simulink model "SimForKid"  (R2019b)
settings: Solver=ode23  StartTime=0.0  StopTime=30  FixedStep=1e-6  RelTol=1e-7
libraries: dsparch4 x3
settings Model: Creator=19398  LastModifiedBy=19398

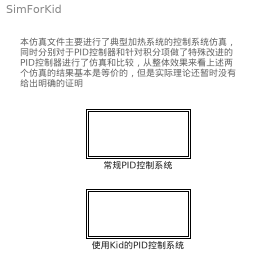
== system SimForKid ==
  note: 本仿真文件主要进行了典型加热系统的控制系统仿真，
      | 同时分别对于PID控制器和针对积分项做了特殊改进的
      | PID控制器进行了仿真和比较，从整体效果来看上述两
      | 个仿真的结果基本是等价的，但是实际理论还暂时没有
      | 给出明确的证明
  使用Kid的PID控制系统 : Subsystem
  常规PID控制系统 : Subsystem

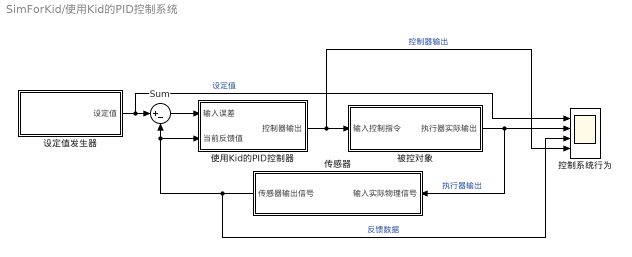
== system SimForKid/使用Kid的PID控制系统 ==
  Sum : Sum  Inputs=|+-
  传感器 : Subsystem
  使用Kid的PID控制器 : Subsystem  mask{Kp=50, Ki=0.5, iLimit=300, Kid=2, Kd=200, c=500, DFilterOrder=6, DFilterFreq=300, OutLim=75}
      mask prompts: Kp "比例增益系数"; Ki "积分增益系数"; iLimit "积分限幅"; Kid "积分微分增益"; Kd "微分增益系数"; c "实际微分系数"; DFilterOrder "微分滤波器阶数"; DFilterFreq "微分滤波器截止频率Hz"; OutLim "输出限幅"
  控制系统行为 : Scope  NumInputPorts=4
  被控对象 : Subsystem
  设定值发生器 : Subsystem
  wires:
  使用Kid的PID控制器/1(控制器输出) -> 控制系统行为/4, 被控对象/1(输入控制指令)  "控制器输出"
  设定值发生器/1(设定值) -> 控制系统行为/1, Sum/1  "设定值"
  被控对象/1(执行器实际输出) -> 控制系统行为/2, 传感器/1(输入实际物理信号)  "执行器输出"
  Sum/1 -> 使用Kid的PID控制器/1(输入误差)
  传感器/1(传感器输出信号) -> 控制系统行为/3, 使用Kid的PID控制器/2(当前反馈值), Sum/2  "反馈数据"

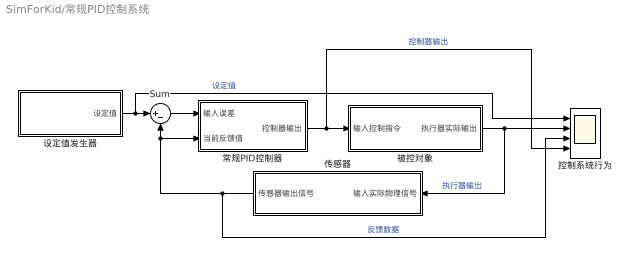
== system SimForKid/常规PID控制系统 ==
  Sum : Sum  Inputs=|+-
  传感器 : Subsystem
  常规PID控制器 : Subsystem  mask{Kp=50, Ki=0.2, iLimit=300, Kd=200, c=500, DFilterOrder=6, DFilterFreq=300, OutLim=75}
      mask prompts: Kp "比例增益系数"; Ki "积分增益系数"; iLimit "积分限幅"; Kd "微分增益系数"; c "实际微分系数"; DFilterOrder "微分滤波器阶数"; DFilterFreq "微分滤波器截止频率Hz"; OutLim "输出限幅"
  控制系统行为 : Scope  NumInputPorts=4
  被控对象 : Subsystem
  设定值发生器 : Subsystem
  wires:
  常规PID控制器/1(控制器输出) -> 控制系统行为/4, 被控对象/1(输入控制指令)  "控制器输出"
  设定值发生器/1(设定值) -> 控制系统行为/1, Sum/1  "设定值"
  被控对象/1(执行器实际输出) -> 控制系统行为/2, 传感器/1(输入实际物理信号)  "执行器输出"
  Sum/1 -> 常规PID控制器/1(输入误差)
  传感器/1(传感器输出信号) -> 控制系统行为/3, 常规PID控制器/2(当前反馈值), Sum/2  "反馈数据"

== system SimForKid/使用Kid的PID控制系统/传感器 ==
  输入实际物理信号 : Inport
  传感滞后 : TransferFcn  Denominator=[6 1]
  通信延迟 : TransportDelay  DelayTime=0.001
  传感器输出信号 : Outport
  wires:
  传感滞后/1 -> 通信延迟/1
  通信延迟/1 -> 传感器输出信号/1
  输入实际物理信号/1 -> 传感滞后/1

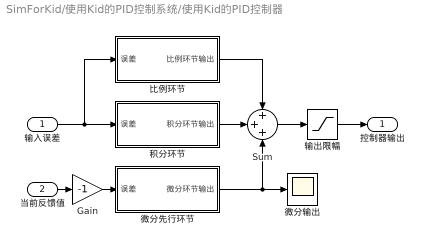
== system SimForKid/使用Kid的PID控制系统/使用Kid的PID控制器 ==
  输入误差 : Inport
  当前反馈值 : Inport  Port=2
  Gain : Gain  Gain=-1
  Sum : Sum  Inputs=+++
  微分先行环节 : Subsystem  mask{Kd=Kd, c=c, DFilterOrder=DFilterOrder, DFilterFreq=DFilterFreq}
      mask prompts: Kd "微分增益系数"; c "实际微分系数"; DFilterOrder "微分滤波器阶数"; DFilterFreq "微分滤波器截止频率Hz"
  微分输出 : Scope
  比例环节 : Subsystem  mask{Kp=Kp}
      mask prompts: Kp "比例增益系数"
  积分环节 : Subsystem  mask{Ki=Ki, iLimit=iLimit, Kid=Kid}
      mask prompts: Ki "积分增益系数"; iLimit "积分限幅"; Kid "积分微分增益"
  输出限幅 : Saturate  UpperLimit=OutLim  LowerLimit=-OutLim  ZeroCross=off
  控制器输出 : Outport
  wires:
  输入误差/1 -> 积分环节/1(误差), 比例环节/1(误差)
  积分环节/1(积分环节输出) -> Sum/2
  比例环节/1(比例环节输出) -> Sum/1
  微分先行环节/1(微分环节输出) -> 微分输出/1, Sum/3
  Sum/1 -> 输出限幅/1
  输出限幅/1 -> 控制器输出/1
  当前反馈值/1 -> Gain/1
  Gain/1 -> 微分先行环节/1(误差)

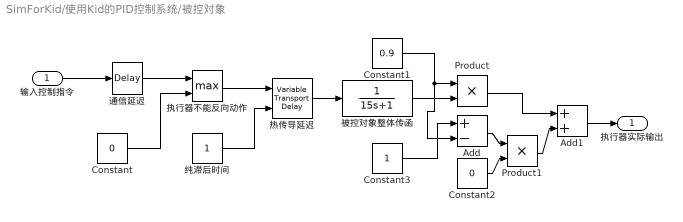
== system SimForKid/使用Kid的PID控制系统/被控对象 ==
  输入控制指令 : Inport
  Add : Sum  Inputs=+-
  Add1 : Sum
  Constant : Constant  Value=0
  Constant1 : Constant  Value=0.9
  Constant2 : Constant  Value=0
  Constant3 : Constant
  Product : Product
  Product1 : Product
  执行器不能反向动作 : MinMax  Function=max  Inputs=2
  热传导延迟 : VariableTransportDelay  MaximumDelay=2
  纯滞后时间 : Constant
  被控对象整体传函 : TransferFcn  Denominator=[15 1]
  通信延迟 : TransportDelay  DelayTime=0.001
  执行器实际输出 : Outport
  wires:
  被控对象整体传函/1 -> Product/2
  输入控制指令/1 -> 通信延迟/1
  通信延迟/1 -> 执行器不能反向动作/1
  Constant/1 -> 执行器不能反向动作/2
  Constant1/1 -> Add/2, Product/1
  Constant3/1 -> Add/1
  Add/1 -> Product1/1
  Constant2/1 -> Product1/2
  Product1/1 -> Add1/2
  Product/1 -> Add1/1
  Add1/1 -> 执行器实际输出/1
  热传导延迟/1 -> 被控对象整体传函/1
  执行器不能反向动作/1 -> 热传导延迟/1
  纯滞后时间/1 -> 热传导延迟/2

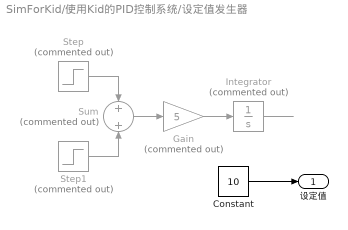
== system SimForKid/使用Kid的PID控制系统/设定值发生器 ==
  Constant : Constant  Value=10
  Gain : Gain  Commented=on  Gain=5
  Integrator : Integrator  Commented=on
  Step : Step  Commented=on  Time=0  SampleTime=0
  Step1 : Step  Commented=on  Time=2  After=-1  SampleTime=0
  Sum : Sum  Commented=on  Inputs=+|+
  设定值 : Outport
  wires:
  Step/1 -> Sum/1
  Step1/1 -> Sum/2
  Gain/1 -> Integrator/1
  Sum/1 -> Gain/1
  Integrator/1 -> ?
  Constant/1 -> 设定值/1

== system SimForKid/常规PID控制系统/传感器 ==
  输入实际物理信号 : Inport
  传感滞后 : TransferFcn  Denominator=[6 1]
  通信延迟 : TransportDelay  DelayTime=0.001
  传感器输出信号 : Outport
  wires:
  传感滞后/1 -> 通信延迟/1
  通信延迟/1 -> 传感器输出信号/1
  输入实际物理信号/1 -> 传感滞后/1

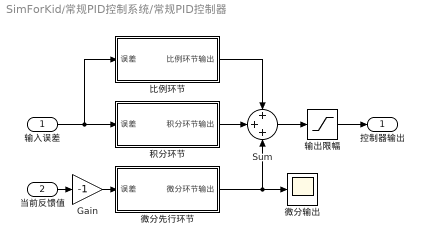
== system SimForKid/常规PID控制系统/常规PID控制器 ==
  输入误差 : Inport
  当前反馈值 : Inport  Port=2
  Gain : Gain  Gain=-1
  Sum : Sum  Inputs=+++
  微分先行环节 : Subsystem  mask{Kd=Kd, c=c, DFilterOrder=DFilterOrder, DFilterFreq=DFilterFreq}
      mask prompts: Kd "微分增益系数"; c "实际微分系数"; DFilterOrder "微分滤波器阶数"; DFilterFreq "微分滤波器截止频率Hz"
  微分输出 : Scope
  比例环节 : Subsystem  mask{Kp=Kp}
      mask prompts: Kp "比例增益系数"
  积分环节 : Subsystem  mask{Ki=Ki, iLimit=iLimit}
      mask prompts: Ki "积分增益系数"; iLimit "积分限幅"
  输出限幅 : Saturate  UpperLimit=OutLim  LowerLimit=-OutLim  ZeroCross=off
  控制器输出 : Outport
  wires:
  输入误差/1 -> 积分环节/1(误差), 比例环节/1(误差)
  积分环节/1(积分环节输出) -> Sum/2
  比例环节/1(比例环节输出) -> Sum/1
  微分先行环节/1(微分环节输出) -> 微分输出/1, Sum/3
  Sum/1 -> 输出限幅/1
  输出限幅/1 -> 控制器输出/1
  当前反馈值/1 -> Gain/1
  Gain/1 -> 微分先行环节/1(误差)

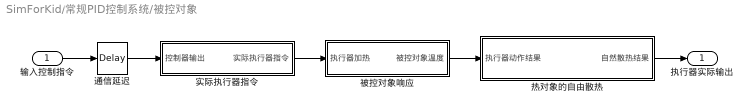
== system SimForKid/常规PID控制系统/被控对象 ==
  输入控制指令 : Inport
  实际执行器指令 : Subsystem
  热对象的自由散热 : Subsystem
  被控对象响应 : Subsystem
  通信延迟 : TransportDelay  DelayTime=0.001
  执行器实际输出 : Outport
  wires:
  输入控制指令/1 -> 通信延迟/1
  通信延迟/1 -> 实际执行器指令/1(控制器输出)
  实际执行器指令/1(实际执行器指令) -> 被控对象响应/1(执行器加热)
  被控对象响应/1(被控对象温度) -> 热对象的自由散热/1(执行器动作结果)
  热对象的自由散热/1(自然散热结果) -> 执行器实际输出/1

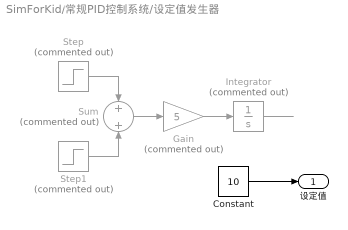
== system SimForKid/常规PID控制系统/设定值发生器 ==
  Constant : Constant  Value=10
  Gain : Gain  Commented=on  Gain=5
  Integrator : Integrator  Commented=on
  Step : Step  Commented=on  Time=0  SampleTime=0
  Step1 : Step  Commented=on  Time=2  After=-1  SampleTime=0
  Sum : Sum  Commented=on  Inputs=+|+
  设定值 : Outport
  wires:
  Step/1 -> Sum/1
  Step1/1 -> Sum/2
  Gain/1 -> Integrator/1
  Sum/1 -> Gain/1
  Integrator/1 -> ?
  Constant/1 -> 设定值/1

== system SimForKid/使用Kid的PID控制系统/使用Kid的PID控制器/微分先行环节 ==
  误差 : Inport
  微分器 : Derivative  CoefficientInTFapproximation=c
  微分增益Kd : Gain  Gain=Kd
  微分滤波器 : dsparch4/Analog Filter Design  method=Butterworth  filttype=Lowpass  N=DFilterOrder  Wlo=2*pi*DFilterFreq  Whi=80  Rp=2  Rs=40
  微分环节输出 : Outport
  wires:
  误差/1 -> 微分增益Kd/1
  微分增益Kd/1 -> 微分滤波器/1
  微分器/1 -> 微分环节输出/1
  微分滤波器/1 -> 微分器/1

== system SimForKid/使用Kid的PID控制系统/使用Kid的PID控制器/比例环节 ==
  误差 : Inport
  比例增益Kp : Gain  Gain=Kp
  比例环节输出 : Outport
  wires:
  误差/1 -> 比例增益Kp/1
  比例增益Kp/1 -> 比例环节输出/1

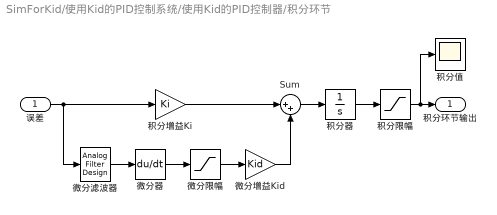
== system SimForKid/使用Kid的PID控制系统/使用Kid的PID控制器/积分环节 ==
  误差 : Inport
  Sum : Sum  Inputs=|++
  微分器 : Derivative  CoefficientInTFapproximation=c
  微分增益Kid : Gain  Gain=Kid
  微分滤波器 : dsparch4/Analog Filter Design  method=Butterworth  filttype=Lowpass  N=DFilterOrder  Wlo=2*pi*DFilterFreq  Whi=80  Rp=2  Rs=40
  微分限幅 : Saturate  UpperLimit=5  LowerLimit=-5
  积分值 : Scope
  积分器 : Integrator
  积分增益Ki : Gain  Gain=Ki
  积分限幅 : Saturate  UpperLimit=iLimit  LowerLimit=-iLimit
  积分环节输出 : Outport
  wires:
  积分器/1 -> 积分限幅/1
  积分限幅/1 -> 积分值/1, 积分环节输出/1
  微分滤波器/1 -> 微分器/1
  误差/1 -> 微分滤波器/1, 积分增益Ki/1
  Sum/1 -> 积分器/1
  积分增益Ki/1 -> Sum/1
  微分器/1 -> 微分限幅/1
  微分限幅/1 -> 微分增益Kid/1
  微分增益Kid/1 -> Sum/2

== system SimForKid/常规PID控制系统/常规PID控制器/微分先行环节 ==
  误差 : Inport
  微分器 : Derivative  CoefficientInTFapproximation=c
  微分增益Kd : Gain  Gain=Kd
  微分滤波器 : dsparch4/Analog Filter Design  method=Butterworth  filttype=Lowpass  N=DFilterOrder  Wlo=2*pi*DFilterFreq  Whi=80  Rp=2  Rs=40
  微分环节输出 : Outport
  wires:
  误差/1 -> 微分增益Kd/1
  微分增益Kd/1 -> 微分滤波器/1
  微分器/1 -> 微分环节输出/1
  微分滤波器/1 -> 微分器/1

== system SimForKid/常规PID控制系统/常规PID控制器/比例环节 ==
  误差 : Inport
  比例增益Kp : Gain  Gain=Kp
  比例环节输出 : Outport
  wires:
  误差/1 -> 比例增益Kp/1
  比例增益Kp/1 -> 比例环节输出/1

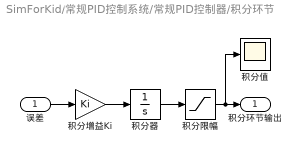
== system SimForKid/常规PID控制系统/常规PID控制器/积分环节 ==
  误差 : Inport
  积分值 : Scope
  积分器 : Integrator
  积分增益Ki : Gain  Gain=Ki
  积分限幅 : Saturate  UpperLimit=iLimit  LowerLimit=-iLimit
  积分环节输出 : Outport
  wires:
  积分器/1 -> 积分限幅/1
  积分限幅/1 -> 积分值/1, 积分环节输出/1
  误差/1 -> 积分增益Ki/1
  积分增益Ki/1 -> 积分器/1

== system SimForKid/常规PID控制系统/被控对象/实际执行器指令 ==
  note: 本仿真中涉及到的控制器只有加热功能而没有散热功能，因而
      | 对于上层控制器给出的负输出结果这里直接取为零
  控制器输出 : Inport
  执行器不能反向动作 : MinMax  Function=max  Inputs=2
  执行器最低输出能力限幅 : Constant  Value=0
  实际执行器指令 : Outport
  wires:
  执行器最低输出能力限幅/1 -> 执行器不能反向动作/2
  控制器输出/1 -> 执行器不能反向动作/1
  执行器不能反向动作/1 -> 实际执行器指令/1

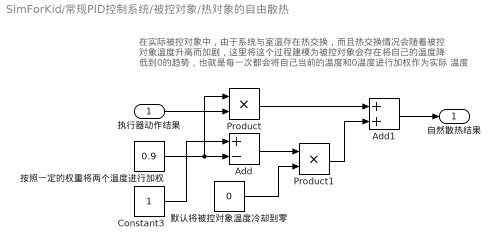
== system SimForKid/常规PID控制系统/被控对象/热对象的自由散热 ==
  note: 在实际被控对象中，由于系统与室温存在热交换，而且热交换情况会随着被控
      | 对象温度升高而加剧，这里将这个过程建模为被控对象会存在将自己的温度降
      | 低到0的趋势，也就是每一次都会将自己当前的温度和0温度进行加权作为实际
      | 温度
  执行器动作结果 : Inport
  Add : Sum  Inputs=+-
  Add1 : Sum
  Constant3 : Constant
  Product : Product
  Product1 : Product
  按照一定的权重将两个温度进行加权 : Constant  Value=0.9
  默认将被控对象温度冷却到零 : Constant  Value=0
  自然散热结果 : Outport
  wires:
  Constant3/1 -> Add/1
  Product/1 -> Add1/1
  Add1/1 -> 自然散热结果/1
  Add/1 -> Product1/1
  执行器动作结果/1 -> Product/2
  Product1/1 -> Add1/2
  按照一定的权重将两个温度进行加权/1 -> Add/2, Product/1
  默认将被控对象温度冷却到零/1 -> Product1/2

== system SimForKid/常规PID控制系统/被控对象/被控对象响应 ==
  note: 这里考虑的加热过程存在纯滞后和惯性滞后两个环节
  执行器加热 : Inport
  热传导延迟 : VariableTransportDelay  MaximumDelay=2
  纯滞后时间 : Constant
  被控对象整体传函 : TransferFcn  Denominator=[15 1]
  被控对象温度 : Outport
  wires:
  纯滞后时间/1 -> 热传导延迟/2
  热传导延迟/1 -> 被控对象整体传函/1
  被控对象整体传函/1 -> 被控对象温度/1
  执行器加热/1 -> 热传导延迟/1
